simulink model "lab2_simulink"  (R2016a)
settings: Solver=VariableStepAuto  StartTime=0.0  StopTime=10.0  MaxStep=0.001  RelTol=1e-3
settings Model: Creator=Karim  LastModifiedBy=Karim

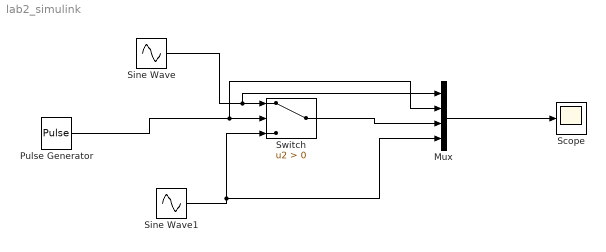
== system lab2_simulink ==
  Mux : Mux
  Pulse Generator : DiscretePulseGenerator  PulseType=Time based  Period=1  PulseWidth=50  PhaseDelay=0.25
  Scope : Scope
  Sine Wave : Sin  SampleTime=0
  Sine Wave1 : Sin  Phase=-pi  Samples=1  SampleTime=0
  Switch : Switch  Criteria=u2 > Threshold
  wires:
  Sine Wave/1 -> Mux/1, Switch/1
  Sine Wave1/1 -> Mux/4, Switch/3
  Pulse Generator/1 -> Mux/2, Switch/2
  Mux/1 -> Scope/1
  Switch/1 -> Mux/3
